simulink model "hh"  (R2018b)
settings: Solver=VariableStepAuto  StartTime=0.0  StopTime=100.0  RelTol=1e-3
undefined symbols (not defined in the file or in its folder): DiscIntNeverNeededParam
libraries: aerolibutil x4, simulink x1, sharedutil x1
settings Model: Creator=Mat  LastModifiedBy=Mat

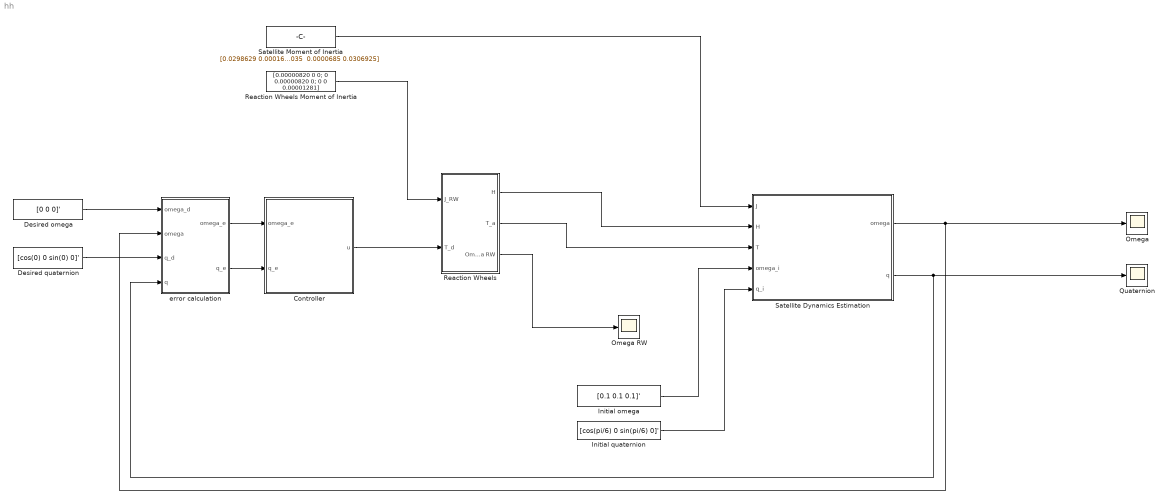
== system hh ==
  Controller : MATLAB Function  TreatAsAtomicUnit=on
  Desired omega : Constant  Value=[0 0 0]'  VectorParams1D=off
  Desired quaternion : Constant  Value=[cos(0) 0 sin(0) 0]'  VectorParams1D=off
  Initial omega : Constant  Value=[0.1 0.1 0.1]'  VectorParams1D=off
  Initial quaternion : Constant  Value=[cos(pi/6) 0 sin(pi/6) 0]'  VectorParams1D=off
  Omega : Scope
  Omega RW : Scope
  Quaternion : Scope
  Reaction Wheels : Subsystem
  Reaction Wheels Moment of Inertia : Constant  Value=|  VectorParams1D=off
      | [0.00000820  0   0;
      |         0   0.00000820  0;
      |         0   0   0.00001281]
  Satellite Dynamics Estimation : Subsystem
  Satellite Moment of Inertia : Constant  Value=|  VectorParams1D=off
      | [0.0298629 0.0001670 0.000035;
      |      0.0001670 0.0063248 0.0000685;
      |      0.000035  0.0000685 0.0306925]
  error calculation : Subsystem
  wires:
  Desired omega/1 -> error calculation/1(omega_d)
  Desired quaternion/1 -> error calculation/3(q_d)
  error calculation/1(omega_e) -> Controller/1(omega_e)
  error calculation/2(q_e) -> Controller/2(q_e)
  Satellite Dynamics Estimation/1(omega) -> error calculation/2("omega "), Omega/1
  Satellite Dynamics Estimation/2(q) -> Quaternion/1, error calculation/4(q)
  Satellite Moment of Inertia/1 -> Satellite Dynamics Estimation/1(J)
  Initial omega/1 -> Satellite Dynamics Estimation/4(omega_i)
  Initial quaternion/1 -> Satellite Dynamics Estimation/5(q_i)
  Reaction Wheels Moment of Inertia/1 -> Reaction Wheels/1(J_RW)
  Controller/1(u) -> Reaction Wheels/2(T_d)
  Reaction Wheels/1(H) -> Satellite Dynamics Estimation/2(H)
  Reaction Wheels/2(T_a) -> Satellite Dynamics Estimation/3(T)
  Reaction Wheels/3(Omega RW) -> Omega RW/1

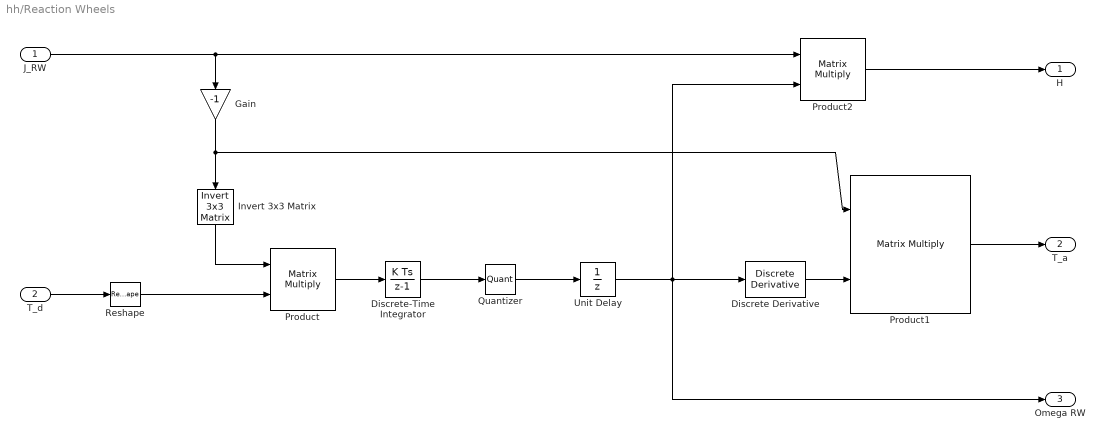
== system hh/Reaction Wheels ==
  J_RW : Inport
  T_d : Inport  Port=2
  Discrete Derivative : simulink/Discrete/Discrete Derivative  gainval=1.0  ICPrevScaledInput=0.0  OutMin=[]  OutMax=[]  OutDataType=fixdt(1, 16)  OutScaling=2^-10  DoSatur=off
  Discrete-Time Integrator : DiscreteIntegrator  SampleTime=-1  ICPrevOutput=DiscIntNeverNeededParam  ICPrevScaledInput=DiscIntNeverNeededParam
  Gain : Gain  Gain=-1
  Invert 3x3 Matrix : aerolibutil/Invert  3x3 Matrix
  Product : Product  Multiplication=Matrix(*)
  Product1 : Product  Multiplication=Matrix(*)
  Product2 : Product  Multiplication=Matrix(*)
  Quantizer : Quantizer  QuantizationInterval=10
  Reshape : Reshape  OutputDimensionality=Column vector (2-D)
  Unit Delay : UnitDelay  SampleTime=0.01
  H : Outport
  T_a : Outport  Port=2
  Omega RW : Outport  Port=3
  wires:
  Discrete Derivative/1 -> Product1/2
  J_RW/1 -> Product2/1, Gain/1
  Discrete-Time Integrator/1 -> Quantizer/1
  Gain/1 -> Invert 3x3 Matrix/1, Product1/1
  Invert 3x3 Matrix/1 -> Product/1
  Reshape/1 -> Product/2
  Product/1 -> Discrete-Time Integrator/1
  T_d/1 -> Reshape/1
  Product1/1 -> T_a/1
  Product2/1 -> H/1
  Quantizer/1 -> Unit Delay/1
  Unit Delay/1 -> Discrete Derivative/1, Product2/2, Omega RW/1

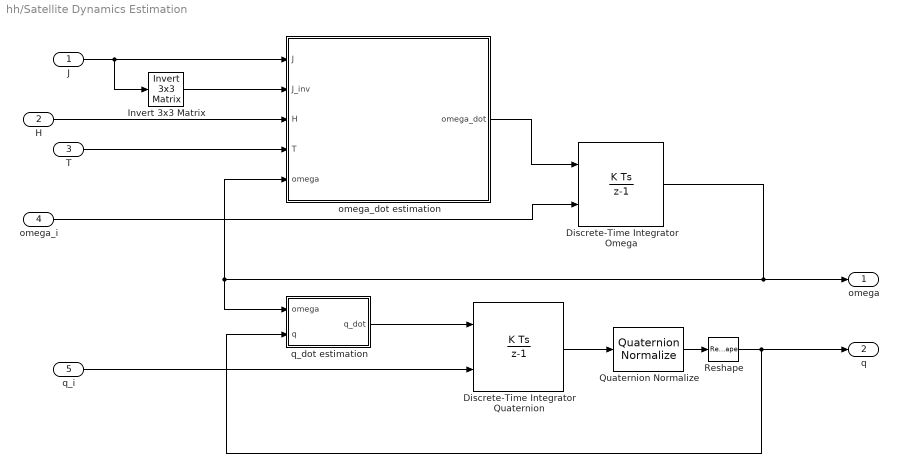
== system hh/Satellite Dynamics Estimation ==
  J : Inport
  H : Inport  Port=2
  T : Inport  Port=3
  omega_i : Inport  Port=4
  q_i : Inport  Port=5
  Discrete-Time Integrator Omega : DiscreteIntegrator  InitialConditionSource=external  SampleTime=-1  ICPrevOutput=DiscIntNeverNeededParam  ICPrevScaledInput=DiscIntNeverNeededParam
  "Discrete-Time Integrator Quaternion " : DiscreteIntegrator  InitialConditionSource=external  SampleTime=-1  ICPrevOutput=DiscIntNeverNeededParam  ICPrevScaledInput=DiscIntNeverNeededParam
  Invert 3x3 Matrix : aerolibutil/Invert  3x3 Matrix
  "Quaternion Normalize " : sharedutil/Quaternion Normalize  aMode=aMode
      settings: SourceProductName=Aerospace Blockset  SourceProductBaseCode=AE
  Reshape : Reshape  OutputDimensionality=Column vector (2-D)
  omega_dot estimation : MATLAB Function  TreatAsAtomicUnit=on
  q_dot estimation : MATLAB Function  TreatAsAtomicUnit=on
  omega : Outport
  q : Outport  Port=2
  wires:
  q_i/1 -> "Discrete-Time Integrator Quaternion "/2
  omega_i/1 -> Discrete-Time Integrator Omega/2
  Invert 3x3 Matrix/1 -> omega_dot estimation/2(J_inv)
  J/1 -> omega_dot estimation/1(J), Invert 3x3 Matrix/1
  q_dot estimation/1(q_dot) -> "Discrete-Time Integrator Quaternion "/1
  "Discrete-Time Integrator Quaternion "/1 -> "Quaternion Normalize "/1
  omega_dot estimation/1(omega_dot) -> Discrete-Time Integrator Omega/1
  Discrete-Time Integrator Omega/1 -> q_dot estimation/1(omega), omega_dot estimation/5(omega), omega/1
  H/1 -> omega_dot estimation/3(H)
  T/1 -> omega_dot estimation/4(T)
  "Quaternion Normalize "/1 -> Reshape/1
  Reshape/1 -> q_dot estimation/2(q), q/1

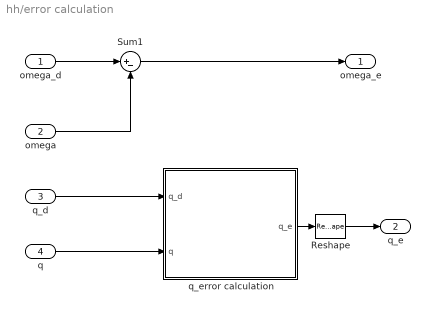
== system hh/error calculation ==
  omega_d : Inport
  "omega " : Inport  Port=2
  q_d : Inport  Port=3
  q : Inport  Port=4
  Reshape : Reshape  OutputDimensionality=Column vector (2-D)
  Sum1 : Sum  Inputs=|+-
  q_error calculation : Subsystem
  omega_e : Outport
  q_e : Outport  Port=2
  wires:
  q_error calculation/1(q_e) -> Reshape/1
  "omega "/1 -> Sum1/2
  q_d/1 -> q_error calculation/1(q_d)
  omega_d/1 -> Sum1/1
  Sum1/1 -> omega_e/1
  q/1 -> q_error calculation/2("q ")
  Reshape/1 -> q_e/1

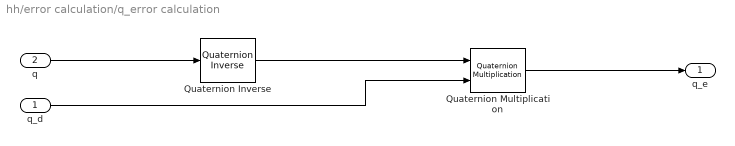
== system hh/error calculation/q_error calculation ==
  q_d : Inport
  "q " : Inport  Port=2
  Quaternion Inverse : aerolibutil/Quaternion Inverse
      settings: SourceProductName=Aerospace Blockset
  Quaternion Multiplication : aerolibutil/Quaternion Multiplication
  q_e : Outport
  wires:
  "q "/1 -> Quaternion Inverse/1
  Quaternion Inverse/1 -> Quaternion Multiplication/1
  q_d/1 -> Quaternion Multiplication/2
  Quaternion Multiplication/1 -> q_e/1

== matlab function hh/Satellite Dynamics Estimation/omega_dot estimation ==
  data: J input; J_inv input; H input; T input; omega_dot output; omega input
function omega_dot = Omega_Dot(J,J_inv,H,T,omega)
cross_omega = [0 -omega(3) omega(2); 
               omega(3) 0 -omega(1); 
              -omega(2) omega(1) 0]; 
omega_dot = J_inv*((-cross_omega*(J*omega+H)) + T);  % From Yang

== matlab function hh/Satellite Dynamics Estimation/q_dot estimation ==
  data: omega input; q_dot output; q input
function q_dot = Q_Dot(omega,q)     % q_dot estimation taken from Yang
sscross_omega = [0 -omega(1) -omega(2) -omega(3); 
                omega(1) 0    omega(3) -omega(2); 
                omega(2) -omega(3) 0    omega(1); 
                omega(3)  omega(2) -omega(1) 0]; 
sscross_q = [q(1) -q(4)  q(3);
             q(4)  q(1) -q(2);
            -q(3)  q(2)  q(1);];
q_dot = 0.5*sscross_omega*q;

== matlab function hh/Controller ==
  data: omega_e input; u output; q_e input
function u = PD(omega_e,q_e)
% This block performs simple PID control with gains:
K_p = 0.1;
K_d = 0.1; % omega_e is assumed directly proportional to q_dot_e

u = K_p*q_e(2:4)*q_e(1) + K_d*omega_e;
